simulink model "power_acdrive"  (Simulink 6.0)
settings: Solver=FixedStepDiscrete  SolverMode=SingleTasking  StartTime=0.0  StopTime=3  RelTol=1e-3
InitFcn:
  | assignin('base','Ts',[2e-6]); load power_acdrive_init;
undefined symbols (not defined in the file or in its folder): DiscIntNeverNeededParam, Ts
libraries: powerlib x5, simulink x2
Description:
  | The Model initialization function Callback automatically
  | 
  | sets the sample time  to 2e-6 sec.  and loads the initial
  | 
  | states vector xInitial. The initial state vector is saved in the
  | 
  | power_acdrive_init.mat file.
  | 
  | 
  | 
  | Check  the Initial state checkbox in the Simulation
  | 
  | parameters/Workspace I/O to start in steady state with a
  | 
  | speed of 120 rad/s and a torque of 0 N.m/s,
settings Model: Creator=Hoang Lehuy, Laval University  LastModifiedBy=batserve  ExtModeTrigMode=oneshot  ExtModeArmWhenConnect=off  ExtModeAutoUpdateStatusClock=off
settings DataIOCC: LimitDataPoints=off  SaveFinalState=on  SaveFormat=StructureWithTime  SaveOutput=off  SaveTime=off  SignalLoggingName=sigsOut
settings OptimizationCC: BlockReduction=off
settings DebuggingCC: CheckExecutionContextPreStartOutputMsg=on  CheckExecutionContextRuntimeOutputMsg=on  SolverPrmCheckMsg=none  UnconnectedOutputMsg=none
settings HardwareCC: TargetUnknown=on
settings RTWCC: TemplateMakefile=grt_vc.tmf

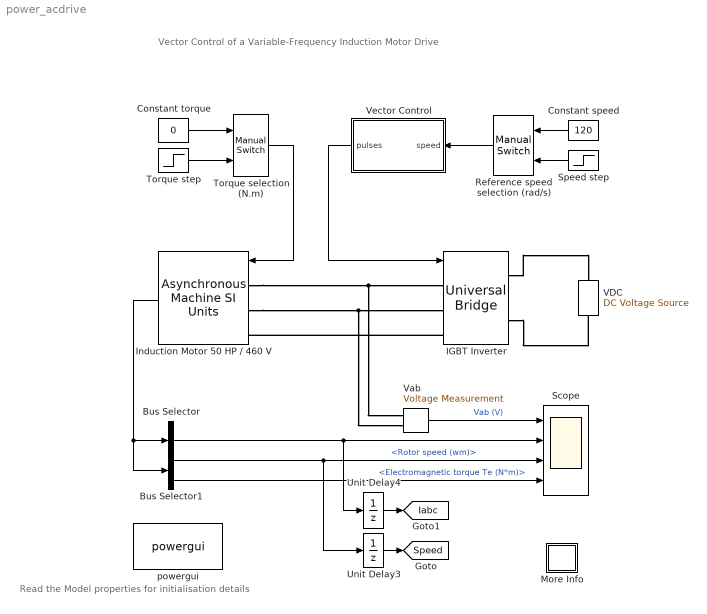
== system power_acdrive ==
  note: Read the Model properties
      | for initialisation details
  note: Vector Control of a Variable-Frequency Induction Motor Drive
  Bus Selector : BusSelector  DialogController=Simulink.DDGSource_Bus  OutputSignals=Stator measurements.Stator current is_a (A),Stator measurements.Stator current is_b (A),Stator measurements.Stator current is_c (A)  MuxedOutput=on
  Bus Selector1 : BusSelector  DialogController=Simulink.DDGSource_Bus  OutputSignals=Mechanical.Rotor speed (wm),Mechanical.Electromagnetic torque Te (N*m)
  Constant speed : Constant  Orientation=left  Value=120
  Constant torque : Constant  Value=0
  IGBT Inverter : powerlib/Power Electronics/Universal Bridge  Arms=3  SnubberResistance=1000  SnubberCapacitance=inf  Device=IGBT / Diodes  Ron=1e-3  Lon=0  ForwardVoltages="[  0.8  0.8  ]"  ForwardVoltage=.8  GTOparameters=[ 1e-6 , 1e-6 ]  IGBTparameters=[ 1e-6 , 2e-6 ]  Measurements=None
  Induction Motor 50 HP / 460 V : powerlib/Machines/Asynchronous Machine SI Units  Orientation=left  PresetModel=No  ShowDetailedParameters=on  RotorType=Squirrel-cage  ReferenceFrame=Stationary  NominalParameters=[ 50*746, 460, 60 ]  Stator=[ 0.087 0.8e-3 ]  Rotor="[ 0.228  0.8e-3 ]"  Lm=34.7e-3  Mechanical="[1.662  0.1 2 ]"  InitialConditions="[ 1, 0 ,  0 , 0 , 0 , 0 , 0 , 0 ]"  Units=1  LoadFlowParameters=0
  More Info : Subsystem
      mask Display: disp('?')
  Reference speed selection (rad/s) : simulink/Signal Routing/Manual Switch  Orientation=left  sw=1  action=0
  Scope : Scope  NumInputPorts=4
      settings: TimeRange=2.5  YMin=-1000~-200~100~-100  YMax=1000~200~180~400  Decimation=20  SampleTime=5e-6
  Speed step : Step  Orientation=left  Time=0.2  Before=120  After=160  SampleTime=0
  Torque selection (N.m) : simulink/Signal Routing/Manual Switch  sw=1  action=0
  Torque step : Step  Time=1.8  After=200  SampleTime=0
  Unit Delay3 : UnitDelay  SampleTime=Ts
  Unit Delay4 : UnitDelay  SampleTime=Ts
  VDC : powerlib/Electrical Sources/DC Voltage Source  Description=source block  Orientation=up  Amplitude=780  Measurements=None
      settings: AttributesFormatString=\n
  Vab : powerlib/Measurements/Voltage Measurement  Tag=PoWeRsYsTeMmEaSuReMeNt  PhasorSimulation=off  OutputType=Magnitude  PSBequivalent=0
  Vector Control : Subsystem  Orientation=left
  powergui : powerlib/powergui  Priority=2  Frange=[0:2:500]  Ylog=off  Xlog=on  save=off  variable=ZData  ZoomFFT=on  StartTime=0.0  cycles=1  DisplayStyle=off  fundamental=60  FreqAxis=off  MaxFrequency=1000  frequencyindice=1  frequencyindicesteady=1  RmsSteady=1  display=off  Ts=Ts  methode=off  frequency=60  echomessages=off
  tag scope: Iabc=global, Speed=global
  wires:
  Bus Selector1/1 -> Unit Delay3/1, Scope/3  "<Rotor speed (wm)>"
  Vector Control/1(pulses) -> IGBT Inverter/1
  Torque step/1 -> Torque selection (N.m)/2
  Constant torque/1 -> Torque selection (N.m)/1
  Constant speed/1 -> Reference speed selection (rad/s)/1
  Speed step/1 -> Reference speed selection (rad/s)/2
  Bus Selector/1 -> Unit Delay4/1, Scope/2
  Unit Delay3/1 -> [Speed]
  Vab/1 -> Scope/1  "Vab (V)"
  Bus Selector1/2 -> Scope/4  "<Electromagnetic torque Te (N*m)>"
  Unit Delay4/1 -> [Iabc]
  Torque selection (N.m)/1 -> Induction Motor 50 HP / 460 V/1
  Reference speed selection (rad/s)/1 -> Vector Control/1(speed)
  Induction Motor 50 HP / 460 V/1 -> Bus Selector1/1, Bus Selector/1
  connections:
  IGBT Inverter/RConn2 -- VDC/LConn1
  IGBT Inverter/LConn3 -- Induction Motor 50 HP / 460 V/LConn3
  Induction Motor 50 HP / 460 V/LConn2 -- IGBT Inverter/LConn2 -- Vab/LConn2
  Induction Motor 50 HP / 460 V/LConn1 -- IGBT Inverter/LConn1 -- Vab/LConn1
  IGBT Inverter/RConn1 -- VDC/RConn1

== system power_acdrive/More Info ==
  note: H. Le-Huy (Universite Laval, Quebec)
  note: 2) In order to reduce the number of points stored in the scope memory, a decimation factor of 20 is used.
  note: 1) The system (control and power sytem) has been discretized with a 2 us time step.
  note: Notes
  note: Case study : Variable-Frequency Induction Motor Drive
  note: Circuit Description
  note: Demonstration
  note: The induction motor is fed by a current-controlled PWM inverter which is built using a Universal Bridge block.
      | The motor drives a mechanical load characterized by inertia J, friction coeficient B, and load torque TL .
      | The speed control loop uses a proportional-integral controller to produce the quadrature-axis current reference
      | iq* which controls the motor torque.  The motor flux is controlled by the direct-axis current reference id*.
      | Block DQ-ABC is used to convert id* and iq* into current references ia*, ib*, and ic* for the current regulator.
      | Current and Voltage Measurement blocks provide signals for visualization purpose.
      | Motor current, speed, and torque signals are available at the output of the 'Asynchronous Machine' block.
  note: Start the simulation. Observe the motor current, voltage, speed, and torque during the starting on the scope.
      |
      | At the end of the simulation time (2.5 s), the system has reached its steady-state. The final state vector can
      | be saved by previously  selecting 'Workspace I/O/Save to workspace/Final state' in Simulation/Parameters window.
      | Once the simultion is finished save the xFinal variable into xInitial.
      |
      | Note : The initial conditions state vector 'xInitial' to start with wm = 120 rad/s and TL = 0 N.m is stored in the
      |             'power_acdrive_init.mat'  file. This  vector is automatically loaded  in your  workspace.
      |
      | Double click the two Manual Switch blocks to switch from  the constant wref and TL blocks to the Step blocks.
      | (Refence speed wref changed from 120 to 160 rad/s at t = 0.2 s and load torque changed from 0 to 200 N.m at  t= 1.4s).
      | In the Simulation/Simulation parameters/Workspace I/O menu, check 'Initial state'  to use the xInitial vector of initial conditions.
      | Restart the simulation  and observe the drive response to successive changes in speed reference and load torque.

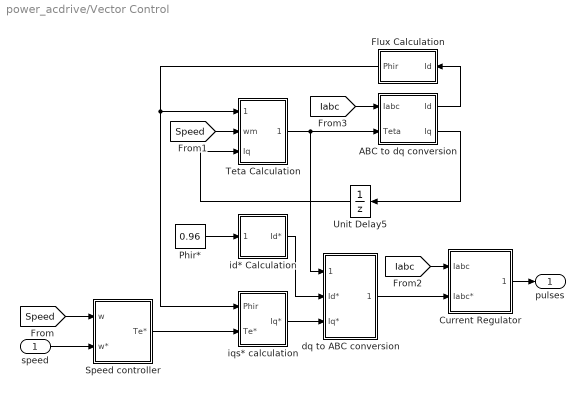
== system power_acdrive/Vector Control ==
  speed : Inport  Port=1  LatchInput=off
  ABC to dq conversion : Subsystem
  Current Regulator : Subsystem  mask(Regulateur de courant a hysteresis){h=20}
      mask prompts: h "Hysteresis band (A)"
  Flux Calculation : Subsystem  Orientation=left  mask(Flux Calcultation){}
      mask init:
      | NF=0.44572610323020e-6;
      | DF=[1 -0.99998715486734];
  Phir* : Constant  Value=0.96
  Speed controller : Subsystem  mask(PI controller){Kp=13, Ki=26, Tlim=300, Ts=Ts}
      mask prompts: Kp "Proportional gain (Kp)"; Ki "Integral gain (Ki)"; Tlim "Torque limit (N.m)"; Ts "Sampling time (s)"
      mask help: Proportional-Integral Speed Controller
      mask Display: plot(0,0,100,100,[35,35,65],[70,30,30],[35,65],[45,60])
  Teta Calculation : Subsystem
  Unit Delay5 : UnitDelay  Orientation=left  SampleTime=Ts
  dq to ABC conversion : Subsystem
  id* Calculation : Subsystem
  iqs* calculation : Subsystem
  pulses : Outport
  wires:
  dq to ABC conversion/1(Iabc*) -> Current Regulator/2(Iabc*)
  Speed controller/1(Te*) -> iqs* calculation/2(Te*)
  Phir*/1 -> id* Calculation/1(Phir*)
  ABC to dq conversion/1(Id) -> Flux Calculation/1(Id)
  id* Calculation/1(Id*) -> dq to ABC conversion/2(Id*)
  Flux Calculation/1(Phir) -> Teta Calculation/1(Phir), iqs* calculation/1(Phir)
  ABC to dq conversion/2(Iq) -> Unit Delay5/1
  Unit Delay5/1 -> Teta Calculation/3(Iq)
  iqs* calculation/1(Iq*) -> dq to ABC conversion/3(Iq*)
  Teta Calculation/1(Teta) -> dq to ABC conversion/1(Teta), ABC to dq conversion/2(Teta)
  [Speed] -> Speed controller/1(w)
  [Speed] -> Teta Calculation/2(wm)
  [Iabc] -> Current Regulator/1(Iabc)
  [Iabc] -> ABC to dq conversion/1(Iabc)
  speed/1 -> Speed controller/2(w*)
  Current Regulator/1(Pulses) -> pulses/1

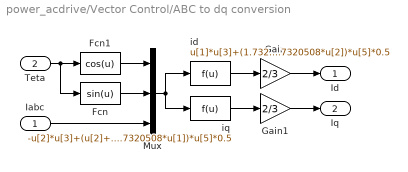
== system power_acdrive/Vector Control/ABC to dq conversion ==
  Iabc : Inport  Port=1  LatchInput=off
  Teta : Inport  Port=2  LatchInput=off
  Fcn : Fcn  Expr=sin(u)
  Fcn1 : Fcn  Expr=cos(u)
  Gain : Gain  Gain=2/3  SaturateOnIntegerOverflow=on
  Gain1 : Gain  Gain=2/3  SaturateOnIntegerOverflow=on
  Mux : Mux  Inputs=[1 1 3]
  id : Fcn  Expr=u[1]*u[3]+(1.7320508*u[2]-u[1])*u[4]*0.5+(-u[1]-1.7320508*u[2])*u[5]*0.5
  iq : Fcn  Expr=-u[2]*u[3]+(u[2]+1.7320508*u[1])*u[4]*0.5+(u[2]-1.7320508*u[1])*u[5]*0.5
  Id : Outport  InitialOutput=0
  Iq : Outport  Port=2  InitialOutput=0
  wires:
  Fcn/1 -> Mux/2
  Fcn1/1 -> Mux/1
  Teta/1 -> Fcn1/1, Fcn/1
  Mux/1 -> iq/1, id/1
  Iabc/1 -> Mux/3
  iq/1 -> Gain1/1
  id/1 -> Gain/1
  Gain/1 -> Id/1
  Gain1/1 -> Iq/1

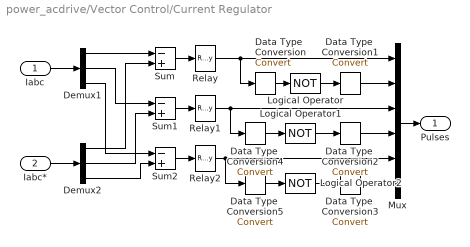
== system power_acdrive/Vector Control/Current Regulator ==
  Iabc : Inport  Port=1  LatchInput=off
  Iabc* : Inport  Port=2  LatchInput=off
  Data Type  Conversion : DataTypeConversion  OutDataTypeMode=boolean  SaturateOnIntegerOverflow=on  RndMeth=Zero
  Data Type  Conversion1 : DataTypeConversion  OutDataTypeMode=double  SaturateOnIntegerOverflow=on  RndMeth=Zero
  Data Type  Conversion2 : DataTypeConversion  OutDataTypeMode=double  SaturateOnIntegerOverflow=on  RndMeth=Zero
  Data Type  Conversion3 : DataTypeConversion  OutDataTypeMode=double  SaturateOnIntegerOverflow=on  RndMeth=Zero
  Data Type  Conversion4 : DataTypeConversion  OutDataTypeMode=boolean  SaturateOnIntegerOverflow=on  RndMeth=Zero
  Data Type  Conversion5 : DataTypeConversion  OutDataTypeMode=boolean  SaturateOnIntegerOverflow=on  RndMeth=Zero
  Demux1 : Demux  Outputs=3
  Demux2 : Demux  Outputs=3
  Logical Operator : Logic  Operator=NOT
  Logical Operator1 : Logic  Operator=NOT
  Logical Operator2 : Logic  Operator=NOT
  Mux : Mux  Inputs=6
  Relay : Relay  OnSwitchValue=h/2  OffSwitchValue=-h/2
  Relay1 : Relay  OnSwitchValue=h/2  OffSwitchValue=-h/2
  Relay2 : Relay  OnSwitchValue=h/2  OffSwitchValue=-h/2
  Sum : Sum  Inputs=-+  SaturateOnIntegerOverflow=on  InputSameDT=on
  Sum1 : Sum  Inputs=-+  SaturateOnIntegerOverflow=on  InputSameDT=on
  Sum2 : Sum  Inputs=-+  SaturateOnIntegerOverflow=on  InputSameDT=on
  Pulses : Outport  InitialOutput=0
  wires:
  Sum/1 -> Relay/1
  Sum1/1 -> Relay1/1
  Demux1/1 -> Sum/1
  Demux1/2 -> Sum1/1
  Mux/1 -> Pulses/1
  Iabc/1 -> Demux1/1
  Sum2/1 -> Relay2/1
  Demux1/3 -> Sum2/1
  Demux2/3 -> Sum2/2
  Demux2/2 -> Sum1/2
  Demux2/1 -> Sum/2
  Iabc*/1 -> Demux2/1
  Relay/1 -> Mux/1, Data Type  Conversion/1
  Relay1/1 -> Mux/3, Data Type  Conversion4/1
  Relay2/1 -> Mux/5, Data Type  Conversion5/1
  Data Type  Conversion/1 -> Logical Operator/1
  Logical Operator/1 -> Data Type  Conversion1/1
  Data Type  Conversion1/1 -> Mux/2
  Logical Operator1/1 -> Data Type  Conversion2/1
  Data Type  Conversion2/1 -> Mux/4
  Logical Operator2/1 -> Data Type  Conversion3/1
  Data Type  Conversion3/1 -> Mux/6
  Data Type  Conversion4/1 -> Logical Operator1/1
  Data Type  Conversion5/1 -> Logical Operator2/1

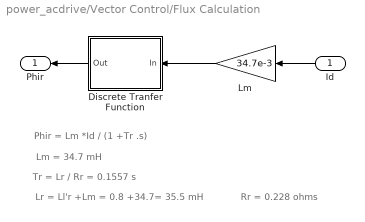
== system power_acdrive/Vector Control/Flux Calculation ==
  note: Phir = Lm *Id / (1 +Tr .s)
  note: Lm = 34.7 mH
  note: Lr = Ll'r +Lm = 0.8 +34.7= 35.5 mH
  note: Tr = Lr / Rr = 0.1557 s
  note: Rr = 0.228 ohms
  Id : Inport  Orientation=left  Port=1  LatchInput=off
  Discrete Tranfer Function : Subsystem  Orientation=left  mask(First Order Low Pass Filter (Discrete)){T=0.1557, Ts=Ts}
      mask prompts: T "Time constant T (s) :"; Ts "Time step (s)"
      mask help: H(s)=1/(1+T.s)
      mask init:
      | X=[0 1 2 3 4];
      |  Y=[-2 -2 -3 -4 -4];
      |  str=sprintf('\nH=1/(1+T.s)\n T= %g s\n\n\n',T);
      | num=1;
      | den=[T 1];
      | 
      | % discrete transfer function
      | % descending powers of z
      | numd= Ts/T;
      | dend=[ 1  (Ts-T)/T];
      mask Display:
      | plot(X,Y);
      | disp(str);
  Lm : Gain  Orientation=left  Gain=34.7e-3  SaturateOnIntegerOverflow=on
  Phir : Outport  Orientation=left
  wires:
  Discrete Tranfer Function/1(Out) -> Phir/1
  Id/1 -> Lm/1
  Lm/1 -> Discrete Tranfer Function/1(In)

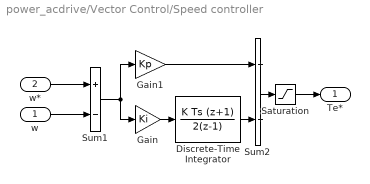
== system power_acdrive/Vector Control/Speed controller ==
  w : Inport  Port=1  LatchInput=off
  w* : Inport  Port=2  LatchInput=off
  Discrete-Time Integrator : DiscreteIntegrator  IntegratorMethod=Integration: Trapezoidal  SampleTime=Ts  LimitOutput=on  UpperSaturationLimit=Tlim  LowerSaturationLimit=-Tlim  ICPrevOutput=DiscIntNeverNeededParam  ICPrevScaledInput=DiscIntNeverNeededParam
  Gain : Gain  Gain=Ki  SaturateOnIntegerOverflow=on
  Gain1 : Gain  Gain=Kp  SaturateOnIntegerOverflow=on
  Saturation : Saturate  UpperLimit=Tlim  LowerLimit=-Tlim
  Sum1 : Sum  Inputs=+-  SaturateOnIntegerOverflow=on  InputSameDT=on
  Sum2 : Sum  SaturateOnIntegerOverflow=on  InputSameDT=on
  Te* : Outport  InitialOutput=0
  wires:
  Gain1/1 -> Sum2/1
  Gain/1 -> Discrete-Time Integrator/1
  Sum1/1 -> Gain/1, Gain1/1
  Discrete-Time Integrator/1 -> Sum2/2
  Sum2/1 -> Saturation/1
  Saturation/1 -> Te*/1
  w/1 -> Sum1/2
  w*/1 -> Sum1/1

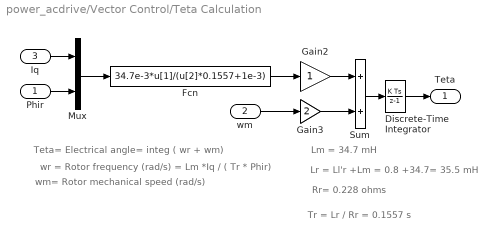
== system power_acdrive/Vector Control/Teta Calculation ==
  note: Teta= Electrical angle= integ ( wr + wm)
  note: wr = Rotor frequency (rad/s) = Lm *Iq / ( Tr * Phir)
  note: Lm = 34.7 mH
  note: Rr= 0.228 ohms
  note: Lr = Ll'r +Lm = 0.8 +34.7= 35.5 mH
  note: wm= Rotor mechanical speed (rad/s)
  note: Tr = Lr / Rr = 0.1557 s
  Phir : Inport  Port=1  LatchInput=off
  wm : Inport  Port=2  LatchInput=off
  Iq : Inport  Port=3  LatchInput=off
  Discrete-Time Integrator : DiscreteIntegrator  SampleTime=Ts  ICPrevOutput=DiscIntNeverNeededParam  ICPrevScaledInput=DiscIntNeverNeededParam
  Fcn : Fcn  Expr=34.7e-3*u[1]/(u[2]*0.1557+1e-3)
  Gain2 : Gain  SaturateOnIntegerOverflow=on
  Gain3 : Gain  Gain=2  SaturateOnIntegerOverflow=on
  Mux : Mux  Inputs=2
  Sum : Sum  SaturateOnIntegerOverflow=on  InputSameDT=on
  Teta : Outport  InitialOutput=0
  wires:
  Discrete-Time Integrator/1 -> Teta/1
  Sum/1 -> Discrete-Time Integrator/1
  Gain3/1 -> Sum/2
  Gain2/1 -> Sum/1
  wm/1 -> Gain3/1
  Fcn/1 -> Gain2/1
  Phir/1 -> Mux/2
  Iq/1 -> Mux/1
  Mux/1 -> Fcn/1

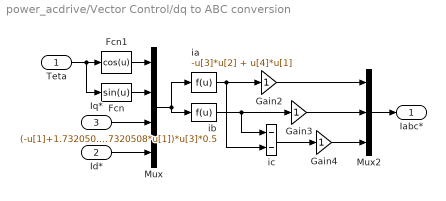
== system power_acdrive/Vector Control/dq to ABC conversion ==
  Teta : Inport  Port=1  LatchInput=off
  Id* : Inport  Port=2  LatchInput=off
  Iq* : Inport  Port=3  LatchInput=off
  Fcn : Fcn  Expr=sin(u)
  Fcn1 : Fcn  Expr=cos(u)
  Gain2 : Gain  SaturateOnIntegerOverflow=on
  Gain3 : Gain  SaturateOnIntegerOverflow=on
  Gain4 : Gain  SaturateOnIntegerOverflow=on
  Mux : Mux
  Mux2 : Mux  Inputs=3
  ia : Fcn  Expr=-u[3]*u[2] + u[4]*u[1]
  ib : Fcn  Expr=(-u[1]+1.7320508*u[2])*u[4]*0.5+(u[2]+1.7320508*u[1])*u[3]*0.5
  ic : Sum  Inputs=--  SaturateOnIntegerOverflow=on  InputSameDT=on
  Iabc* : Outport  InitialOutput=0
  wires:
  Fcn/1 -> Mux/2
  Fcn1/1 -> Mux/1
  Mux2/1 -> Iabc*/1
  Mux/1 -> ib/1, ia/1
  Teta/1 -> Fcn1/1, Fcn/1
  Iq*/1 -> Mux/3
  Id*/1 -> Mux/4
  Gain3/1 -> Mux2/2
  ic/1 -> Gain4/1
  Gain4/1 -> Mux2/3
  Gain2/1 -> Mux2/1
  ia/1 -> Gain2/1, ic/2
  ib/1 -> Gain3/1, ic/1

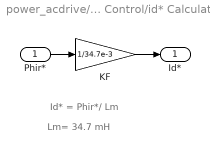
== system power_acdrive/Vector Control/id* Calculation ==
  note: Id* = Phir*/ Lm
  note: Lm= 34.7 mH
  Phir* : Inport  Port=1  LatchInput=off
  KF : Gain  Gain=1/34.7e-3  SaturateOnIntegerOverflow=on
  Id* : Outport
  wires:
  KF/1 -> Id*/1
  Phir*/1 -> KF/1

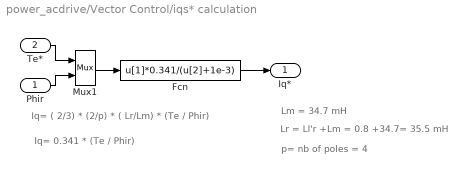
== system power_acdrive/Vector Control/iqs* calculation ==
  note: Iq= ( 2/3) * (2/p) * ( Lr/Lm) * (Te / Phir)
  note: Lm = 34.7 mH
  note: Lr = Ll'r +Lm = 0.8 +34.7= 35.5 mH
  note: p= nb of poles = 4
  note: Iq= 0.341 * (Te / Phir)
  Phir : Inport  Port=1  LatchInput=off
  Te* : Inport  Port=2  LatchInput=off
  Fcn : Fcn  Expr=u[1]*0.341/(u[2]+1e-3)
  Mux1 : Mux  Inputs=2
  Iq* : Outport  InitialOutput=0
  wires:
  Phir/1 -> Mux1/2
  Fcn/1 -> Iq*/1
  Te*/1 -> Mux1/1
  Mux1/1 -> Fcn/1

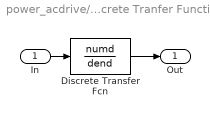
== system power_acdrive/Vector Control/Flux Calculation/Discrete Tranfer Function ==
  In : Inport  Port=1  LatchInput=off
  Discrete Transfer Fcn : DiscreteTransferFcn  Numerator=numd  Denominator=dend  SampleTime=Ts
  Out : Outport  InitialOutput=0
  wires:
  Discrete Transfer Fcn/1 -> Out/1
  In/1 -> Discrete Transfer Fcn/1
